simulink model "fileSimulink"  (R2014a)
settings: Solver=ode45  StartTime=0.0  StopTime=10  RelTol=1e-3
libraries: cstblocks x3, simulink x1
settings Model: Creator=User  LastModifiedBy=User

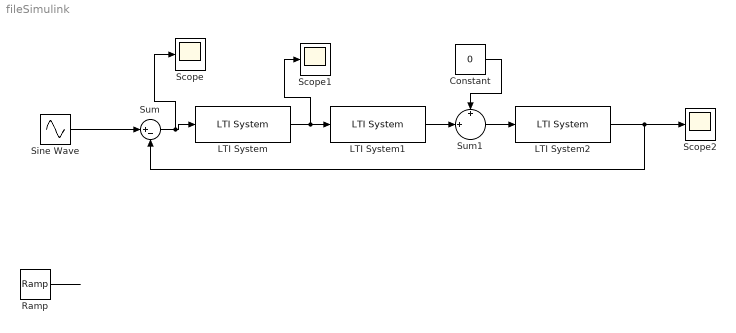
== system fileSimulink ==
  Constant : Constant  Value=0
  LTI System : cstblocks/LTI System  sys=C  IC=[]
  LTI System1 : cstblocks/LTI System  sys=F1  IC=[]
  LTI System2 : cstblocks/LTI System  sys=F2  IC=[]
  Ramp : simulink/Sources/Ramp  slope=0  start=0  X0=0
  Scope : Scope
  Scope1 : Scope
  Scope2 : Scope
      settings: SaveName=ScopeData2
  Sine Wave : Sin  Frequency=0.5  SampleTime=0
  Sum : Sum  Inputs=|+-
  Sum1 : Sum  Inputs=+|+||
  wires:
  LTI System2/1 -> Sum/2, Scope2/1
  LTI System/1 -> Scope1/1, LTI System1/1
  LTI System1/1 -> Sum1/2
  Sum1/1 -> LTI System2/1
  Ramp/1 -> ?
  Sine Wave/1 -> Sum/1
  Sum/1 -> Scope/1, LTI System/1
  Constant/1 -> Sum1/1
